simulink model "schemaSimulink_PD"  (R2016a)
settings: Solver=ode45  StartTime=0.0  StopTime=400  RelTol=1e-3
libraries: fuzblock x1
settings Model: Creator=Ana  LastModifiedBy=Dascalu Ionelia
settings DataIOCC: LimitDataPoints=on  SaveFormat=Array
settings DebuggingCC: UnderspecifiedInitializationDetection=Classic  MergeDetectMultiDrivingBlocksExec=none  SolverPrmCheckMsg=warning  StateNameClashWarn=warning
settings HardwareCC: ProdBitPerPointer=32  ProdLargestAtomicFloat=None  ProdIntDivRoundTo=Undefined  ProdEndianess=Unspecified  ProdWordSize=32  ProdHWDeviceType=32-bit Generic
settings ModelReferenceCC: PropagateSignalLabelsOutOfModel=off
settings ConfigComp: CovModelRefEnable=Off

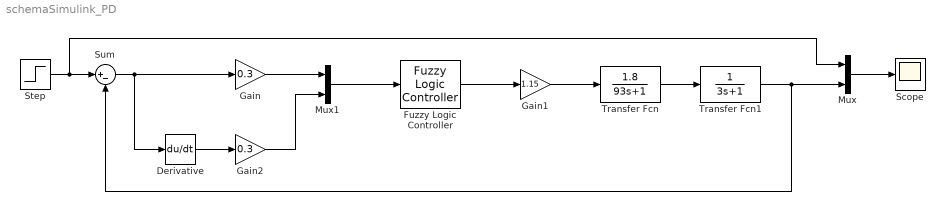
== system schemaSimulink_PD ==
  Derivative : Derivative
  Fuzzy Logic Controller : fuzblock/Fuzzy Logic  Controller  fis=Regulator_PD1
  Gain : Gain  Gain=0.3
  Gain1 : Gain  Gain=1.15
  Gain2 : Gain  Gain=0.3
  Mux : Mux  Inputs=2
  Mux1 : Mux  Inputs=2
  Scope : Scope
  Step : Step  Time=0  SampleTime=0
  Sum : Sum  Inputs=|+-
  Transfer Fcn : TransferFcn  Numerator=[1.8]  Denominator=[93 1]
  Transfer Fcn1 : TransferFcn  Denominator=[3 1]
  wires:
  Sum/1 -> Derivative/1, Gain/1
  Step/1 -> Mux/1, Sum/1
  Derivative/1 -> Gain2/1
  Gain/1 -> Mux1/1
  Gain2/1 -> Mux1/2
  Mux1/1 -> Fuzzy Logic Controller/1
  Fuzzy Logic Controller/1 -> Gain1/1
  Gain1/1 -> Transfer Fcn/1
  Mux/1 -> Scope/1
  Transfer Fcn/1 -> Transfer Fcn1/1
  Transfer Fcn1/1 -> Sum/2, Mux/2
